simulink model "DesignTemperatureControlForDataCenter"  (R2025b)
settings: Solver=daessc  StartTime=0.0  StopTime=3600*4  FixedStep=0.5  MaxStep=1  RelTol=1e-3  AbsTol=1e-3
PreLoadFcn:
  | if ~exist("modelParam")
  |     setDefaultParameters;
  | end
undefined symbols (not defined in the file or in its folder): DiscIntNeverNeededParam, modelParam, value
libraries: fl_lib x78, nesl_utility x18, SimscapeFluids_lib x11, datacenter_lib x9, simulink_extras x4, slpidlib x2
(part 2 of 3)

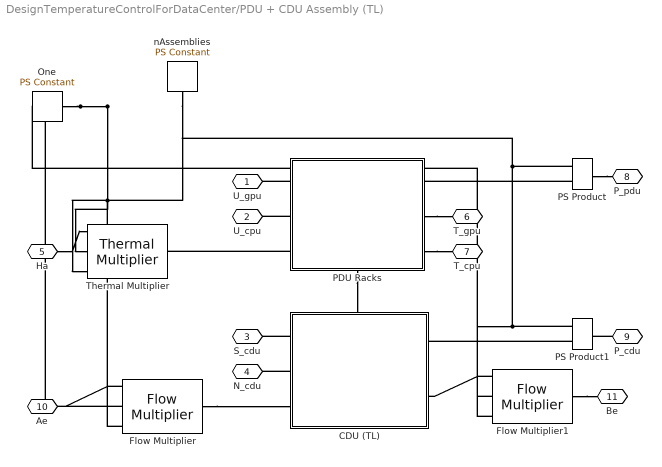
== system DesignTemperatureControlForDataCenter/PDU + CDU Assembly (TL) ==
  CDU (TL) : Subsystem  mask{extFluidMdot=extFluidMdot, extFluidPrDrop=extFluidPrDrop, extFluidVol=extFluidVol, extFluidPipeArea=extFluidPipeArea, intFluidMdot=intFluidMdot, intFluidPrDrop=intFluidPrDrop, intFluidVol=intFluidVol, intFluidPipeArea=intFluidPipeArea, spDissipationTbl=spDissipationTbl, effPipeLen=effPipeLen, pumpCapacityVec=pumpCapacityVec, pumpRefHeadVec=pumpRefHeadVec, pumpRefBrkPowVec=pumpRefBrkPowVec, pumpEff=pumpEff, nPumps=nPumps, speedLimFactor=speedLimFactor, pumpNominalRPM=pumpNominalRPM, pumpImpellerDiaFactor=pumpImpellerDiaFactor, iniT=initialT, iniP=initialP, refT=refT, refP=refP, refDensity=refDensity}
      mask prompts: extFluidMdot "External liquid loop mass flow rate vector (kg/s)"; extFluidPrDrop "External liquid loop pressure drop vector (kPa)"; extFluidVol "External liquid volume in heat exchanger (m^3)"; extFluidPipeArea "External liquid loop pipe cross-sectional area (m^2)"; intFluidMdot "Internal liquid loop mass flow rate vector (kg/s)"; intFluidPrDrop "Internal liquid loop pressure drop vector (kPa)"; intFluidVol "Internal liquid volume in heat exchanger (m^3)"; intFluidPipeArea "Internal liquid loop pipe cross-sectional area (m^2)"; spDissipationTbl "Specific dissipation table, SD[mdot_int,mdot_ext] (kW/K)"; effPipeLen "Effective pipe length for rack cooling (m)"; pumpCapacityVec "Reference capacity vector for each pump (m^3/s)"; pumpRefHeadVec "Reference head vector for each pump (m)"; pumpRefBrkPowVec "Reference brake power vector (kW)"; pumpEff "Electrical efficiency vector, 0-1 (-)"; nPumps "Total number of pumps (-)"; speedLimFactor "Pump speed upper limit factor (-)"; pumpNominalRPM "Pump nominal rating (rpm)"; pumpImpellerDiaFactor "Impeller diameter scale factor (-)"; iniT "Initial temperature (K)"; iniP "Initial pressure (MPa)"; refT "Reference flow temperature (K)"; refP "Reference flow pressure (MPa)"; refDensity "Reference density for internal liquid (kg/m^3)"
      settings: CopyFcn=set_param(gcbh,'LinkStatus','none');  PortSchema="{\"entries\":[{\"content\":{\"sides\":[{\"content\":{\"connectorIds\":[\"LConn1\",\"LConn2\",\"LConn3\"]},\"type\":\"ConnectorPlacement.EquallySpacedRectSide\",\"uuid\":\"dd9276e8-a048-49df-a05c-f18b45aafce3\"},{\"content\":{\"connectorIds\":[\"RConn1\",\"RConn2\"],\"side\":\"RIGHT\"},\"type\":\"ConnectorPlacement.EquallySpacedRectSide\",\"uuid\":\"f4cbe01b-cfd4-4d60-aff7-a07955033ed5\"},{\"content\":{\"connectorIds\":[\"LConn4\"],\"side\":\"TOP\"},\"type\":\"ConnectorPlacement.EquallySpacedRectSide\",\"uuid\":\"ad27df56-4241-452c-8570-6a66062dd2f2\"}]},\"type\":\"ConnectorPlacement.EquallySpacedConnector\",\"uuid\":\"0333b5f9-1896-45e0-922d-790b0e5dd980\"}],\"packageUris\":[\"http://schema.mathworks.com/mf0/Connector/R2020b\"],\"version\":\"1.0\"}"
      mask Help: web("DocumentationCDUTL.html")
      mask DialogControl Container5 Prompt: Heat Exchanger
      mask DialogControl Container8 Prompt: Set External Fluid Properties
      mask DialogControl Container7 Prompt: Set Internal Fluid Properties
      mask DialogControl Container9 Prompt: Heat Transfer
      mask DialogControl Container6 Prompt: Pumps
      mask DialogControl Container4 Prompt: Initial Conditions
      mask Display: image('icon_CDUthermalLiquid.png');
  Flow Multiplier : datacenter_lib/Flow Multiplier
      settings: InternalSimscapePortConfiguration="{\"Bottom\":[],\"Left\":[{\"id\":\"A\",\"label\":\"A\",\"type\":\"foundation.thermal_liquid.thermal_liquid\"}],\"Right\":[{\"id\":\"B\",\"label\":\"B\",\"type\":\"foundation.thermal_liquid.thermal_liquid\"}],\"Top\":[{\"id\":\"Na\",\"label\":\"Na\",\"type\":\"input\"},{\"id\":\"Nb\",\"label\":\"Nb\",\"type\":\"input\"}]}"
  Flow Multiplier1 : datacenter_lib/Flow Multiplier
      settings: InternalSimscapePortConfiguration="{\"Bottom\":[],\"Left\":[{\"id\":\"A\",\"label\":\"A\",\"type\":\"foundation.thermal_liquid.thermal_liquid\"}],\"Right\":[{\"id\":\"B\",\"label\":\"B\",\"type\":\"foundation.thermal_liquid.thermal_liquid\"}],\"Top\":[{\"id\":\"Na\",\"label\":\"Na\",\"type\":\"input\"},{\"id\":\"Nb\",\"label\":\"Nb\",\"type\":\"input\"}]}"
  One : fl_lib/Physical Signals/Sources/PS Constant  constant=1
  PDU Racks : Subsystem  mask{nTrays=nTrays, nRacks=nRacks, trayMass=trayMass, trayCp=trayCp, trayThermalR=trayThermalR, nGPU=nGPU, gpuTDPperDie=gpuTDPperDie, gpuIdlePower=gpuIdlePower, gpuHBMpower=gpuHBMpower, gpuExponent=gpuExponent, gpuHBMutil=gpuHBMutil, gpuLeakage=gpuLeakage, gpuNominalDieT=gpuNominalDieT, gpuDieThermalC=gpuDieThermalC, gpuHeatSinkR=gpuHeatSinkR, gpuSurfArea=gpuSurfArea, gpuAmbientR=gpuAmbientR, nCPU=nCPU, cpuTDPperSocket=cpuTDPperSocket, cpuIdlePower=cpuIdlePower, cpuExponent=cpuExponent, cpuLeakage=cpuLeakage, cpuNominalDieT=cpuNominalDieT, cpuDieThermalC=cpuDieThermalC, cpuHeatSinkR=cpuHeatSinkR, cpuSurfArea=cpuSurfArea, cpuAmbientR=cpuAmbientR, initialT=initialT, htc=htc}
      mask prompts: nTrays "Number of IT trays per rack (-)"; nRacks "Number of racks (-)"; trayMass "Tray mass (kg)"; trayCp "Tray specific heat capacity (J/kg*K)"; trayThermalR "Tray to external thermal resistance (K/W)"; nGPU "Number of GPU per tray (-)"; gpuTDPperDie "GPU TDP per die (W)"; gpuIdlePower "GPU idle power (W)"; gpuHBMpower "HBM power per GPU (W)"; gpuExponent "GPU power utilization exponent (-)"; gpuHBMutil "HBM utilization as fraction of compute utilization (-)"; gpuLeakage "Leakage increase per K above nominal temperature (W/K)"; gpuNominalDieT "Nominal die temperature at TDP (K)"; gpuDieThermalC "GPU die thermal capacitance (J/K)"; gpuHeatSinkR "GPU die-heat-sink thermal resistance (K/W)"; gpuSurfArea "Surface area per die for ambient heat transfer (m^2)"; gpuAmbientR "GPU die-ambient thermal resistance (K/W)"; nCPU "Number of CPU per tray (-)"; cpuTDPperSocket "CPU TDP per socket (W)"; cpuIdlePower "CPU idle power per socket (W)"; cpuExponent "CPU power utilization exponent (-)"; cpuLeakage "Leakage increase per K above nominal temperature (W/K)"; cpuNominalDieT "Nominal die temperature at TDP (K)"; cpuDieThermalC "CPU die thermal capacitance (J/K)"; cpuHeatSinkR "CPU die-heat-sink thermal resistance (K/W)"; cpuSurfArea "Surface area per die for ambient heat transfer (m^2)"; cpuAmbientR "CPU die-ambient thermal resistance (K/W)"; initialT "Initial temperature (K)"; htc "Heat transfer coefficient to ambient (W/m^2.K)"
      settings: CopyFcn=set_param(gcbh,'LinkStatus','none');  PortSchema="{\"entries\":[{\"content\":{\"sides\":[{\"content\":{\"connectorIds\":[\"LConn1\",\"LConn2\",\"LConn3\"]},\"type\":\"ConnectorPlacement.EquallySpacedRectSide\",\"uuid\":\"1a9a884a-dab1-4495-bf62-c6b2de6c1039\"},{\"content\":{\"connectorIds\":[\"RConn1\",\"RConn2\",\"RConn3\"],\"side\":\"RIGHT\"},\"type\":\"ConnectorPlacement.EquallySpacedRectSide\",\"uuid\":\"05c53434-51c1-4fee-b885-c321dcda8b6b\"},{\"content\":{\"side\":\"TOP\"},\"type\":\"ConnectorPlacement.EquallySpacedRectSide\",\"uuid\":\"c7b5c534-d596-4858-a133-27f005e6c9d4\"},{\"content\":{\"connectorIds\":[\"RConn4\"],\"side\":\"BOTTOM\"},\"type\":\"ConnectorPlacement.EquallySpacedRectSide\",\"uuid\":\"693f3c99-4296-4d86-bfcc-da753d3e576f\"}]},\"type\":\"ConnectorPlacement.EquallySpacedConnector\",\"uuid\":\"ed91c467-c4d0-403f-af16-bac0257594fd\"}],\"packageUris\":[\"http://schema.mathworks.com/mf0/Connector/R2020b\"],\"version\":\"1.0\"}"
      mask Help: web("DocumentationPDURacks.html")
      mask DialogControl Container10 Prompt: PDU Racks
      mask DialogControl getRatingButton Prompt: Get Rating
      mask DialogControl Container9 Prompt: IT Tray
      mask DialogControl Container6 Prompt: GPU
      mask DialogControl Container7 Prompt: CPU
      mask DialogControl Container8 Prompt: Initial Conditions
      mask Display: image('icon_PDURacks.png');
  PS Product : fl_lib/Physical Signals/Functions/PS Product
  PS Product1 : fl_lib/Physical Signals/Functions/PS Product
  Thermal Multiplier : datacenter_lib/Thermal Multiplier
      settings: InternalSimscapePortConfiguration="{\"Bottom\":[],\"Left\":[{\"id\":\"A\",\"label\":\"A\",\"type\":\"foundation.thermal.thermal\"}],\"Right\":[{\"id\":\"B\",\"label\":\"B\",\"type\":\"foundation.thermal.thermal\"}],\"Top\":[{\"id\":\"Na\",\"label\":\"Na\",\"type\":\"input\"},{\"id\":\"Nb\",\"label\":\"Nb\",\"type\":\"input\"}]}"
  nAssemblies : fl_lib/Physical Signals/Sources/PS Constant  constant=nAssembly
  U_gpu : PMIOPort  Side=Left
  U_cpu : PMIOPort  Port=2  Side=Left
  S_cdu : PMIOPort  Port=3  Side=Left
  N_cdu : PMIOPort  Port=4  Side=Left
  Ha : PMIOPort  Port=5  Side=Left
  T_gpu : PMIOPort  Port=6  Side=Right
  T_cpu : PMIOPort  Port=7  Side=Right
  P_pdu : PMIOPort  Port=8  Side=Right
  P_cdu : PMIOPort  Port=9  Side=Right
  Ae : PMIOPort  Port=10  Side=Right
  Be : PMIOPort  Port=11  Side=Right
  connections:
  P_cdu/RConn1 -- PS Product1/RConn1
  PS Product1/LConn2 -- CDU (TL)/RConn1
  PS Product/RConn1 -- P_pdu/RConn1
  PS Product/LConn2 -- PDU Racks/RConn1
  Flow Multiplier/LConn3 -- Thermal Multiplier/LConn3 -- PS Product/LConn1 -- Flow Multiplier1/LConn2 -- PS Product1/LConn1 -- nAssemblies/RConn1
  Thermal Multiplier/LConn2 -- Flow Multiplier1/LConn3 -- Flow Multiplier/LConn2 -- One/RConn1
  Flow Multiplier1/LConn1 -- CDU (TL)/RConn2
  Flow Multiplier1/RConn1 -- Be/RConn1
  Flow Multiplier/RConn1 -- CDU (TL)/LConn3
  Flow Multiplier/LConn1 -- Ae/RConn1
  Ha/RConn1 -- Thermal Multiplier/LConn1
  PDU Racks/LConn3 -- Thermal Multiplier/RConn1
  CDU (TL)/LConn1 -- S_cdu/RConn1
  PDU Racks/LConn1 -- U_gpu/RConn1
  PDU Racks/RConn2 -- T_gpu/RConn1
  CDU (TL)/LConn2 -- N_cdu/RConn1
  PDU Racks/LConn2 -- U_cpu/RConn1
  PDU Racks/RConn3 -- T_cpu/RConn1
  PDU Racks/RConn4 -- CDU (TL)/LConn4

== system DesignTemperatureControlForDataCenter/Pipe ==
  CDU External Water : SimscapeFluids_lib/Thermal Liquid/Utilities/Thermal Liquid Properties (TL)  fluid_list=fluids.thermal_liquid.utilities.enum.thermal_liquid_fluid_list.water  concentration_param_EG=fluids.thermal_liquid.utilities.enum.thermal_liquid_concentration.volume_fraction  concentration_param_PG=fluids.thermal_liquid.utilities.enum.thermal_liquid_concentration.volume_fraction  c_mass_SW=3.5e-3  c_mass_EG=0.1  c_mass_PG=0.1  c_mass_GL=0.1  c_vol_EG=0.1  c_vol_PG=0.1  beta_const_EG=2.1791 GPa  beta_const_PG=2.1791 GPa  beta_const_GL=2.1791 GPa  p_min_EG=0.01 MPa  p_min_PG=0.01 MPa  p_min_GL=0.01 MPa  p_max_EG=50 MPa  p_max_PG=50 MPa  p_max_GL=50 MPa  p_atm=0.101325 MPa  properties_range_check=simscape.enum.assert.action.error
  Perfect Insulator2 : fl_lib/Thermal/Thermal Elements/Perfect Insulator  T_specify=off  T_priority=None  T=293.15 K  T_nominal_specify=off  T_nominal_value=1  T_nominal_unit=K
  Pipe (TL)1 : fl_lib/Thermal Liquid/Elements/Pipe (TL)  length=.1 m  area=0.01*10 m^2  Dh=sqrt((4/pi)*0.01*10) m  length_add=1 m  roughness=15e-6 m  Re_lam=2000  Re_tur=4000  shape_factor=64  Nu_lam=3.66  dynamic_compressibility=true  inertia=false  p0=0.101325 MPa  T0="max(274,value(modelParam.WetBulbT ,\"K\")) K"  mdot0=0 kg/s  p_nominal=0.101325 MPa  T_nominal=293.15 K
  A : PMIOPort  Side=Left
  B : PMIOPort  Port=2  Side=Right
  connections:
  Perfect Insulator2/LConn1 -- Pipe (TL)1/LConn2
  A/RConn1 -- Pipe (TL)1/LConn1
  B/RConn1 -- CDU External Water/RConn1 -- Pipe (TL)1/RConn1

== system DesignTemperatureControlForDataCenter/Pipe  ==
  Cooling Tower Water : SimscapeFluids_lib/Thermal Liquid/Utilities/Thermal Liquid Properties (TL)  fluid_list=fluids.thermal_liquid.utilities.enum.thermal_liquid_fluid_list.water  concentration_param_EG=fluids.thermal_liquid.utilities.enum.thermal_liquid_concentration.volume_fraction  concentration_param_PG=fluids.thermal_liquid.utilities.enum.thermal_liquid_concentration.volume_fraction  c_mass_SW=3.5e-3  c_mass_EG=0.1  c_mass_PG=0.1  c_mass_GL=0.1  c_vol_EG=0.1  c_vol_PG=0.1  beta_const_EG=2.1791 GPa  beta_const_PG=2.1791 GPa  beta_const_GL=2.1791 GPa  p_min_EG=0.01 MPa  p_min_PG=0.01 MPa  p_min_GL=0.01 MPa  p_max_EG=50 MPa  p_max_PG=50 MPa  p_max_GL=50 MPa  p_atm=0.101325 MPa  properties_range_check=simscape.enum.assert.action.error
  Perfect Insulator3 : fl_lib/Thermal/Thermal Elements/Perfect Insulator  T_specify=off  T_priority=None  T=293.15 K  T_nominal_specify=off  T_nominal_value=1  T_nominal_unit=K
  Pipe (TL) : fl_lib/Thermal Liquid/Elements/Pipe (TL)  length=.1 m  area=0.01*10 m^2  Dh=sqrt((4/pi)*0.01*10) m  length_add=1 m  roughness=15e-6 m  Re_lam=2000  Re_tur=4000  shape_factor=64  Nu_lam=3.66  dynamic_compressibility=true  inertia=false  p0=0.101325 MPa  T0="max(274,value(modelParam.WetBulbT ,\"K\")) K"  mdot0=0 kg/s  p_nominal=0.101325 MPa  T_nominal=293.15 K
  A : PMIOPort  Side=Left
  B : PMIOPort  Port=2  Side=Right
  connections:
  Perfect Insulator3/LConn1 -- Pipe (TL)/LConn2
  Pipe (TL)/RConn1 -- Cooling Tower Water/RConn1 -- B/RConn1
  Pipe (TL)/LConn1 -- A/RConn1

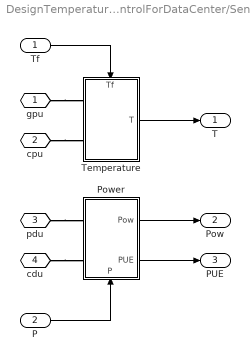
== system DesignTemperatureControlForDataCenter/Sensor ==
  Tf : Inport
  P : Inport  Port=2
  Power : Subsystem
      settings: PortSchema="{\"entries\":[{\"content\":{\"sides\":[{\"content\":{\"connectorIds\":[\"LConn1\",\"LConn2\"]},\"type\":\"ConnectorPlacement.EquallySpacedRectSide\",\"uuid\":\"9331510c-a4eb-4ecd-92c7-a7bb9d97a600\"},{\"content\":{\"connectorIds\":[\"Out1\",\"Out2\"],\"side\":\"RIGHT\"},\"type\":\"ConnectorPlacement.EquallySpacedRectSide\",\"uuid\":\"a10f6118-0032-4cdc-99b8-d09e72885979\"},{\"content\":{\"side\":\"TOP\"},\"type\":\"ConnectorPlacement.EquallySpacedRectSide\",\"uuid\":\"0f2ace20-053e-4299-9751-41cfaf8e15c6\"},{\"content\":{\"connectorIds\":[\"In1\"],\"side\":\"BOTTOM\"},\"type\":\"ConnectorPlacement.EquallySpacedRectSide\",\"uuid\":\"a9d7e431-b1c5-4489-9883-492d0aaca8bd\"}]},\"type\":\"ConnectorPlacement.EquallySpacedConnector\",\"uuid\":\"b3630bca-808a-4a4c-ac99-f11c77996374\"}],\"packageUris\":[\"http://schema.mathworks.com/mf0/Connector/R2020b\"],\"version\":\"1.0\"}"
  Temperature : Subsystem
      settings: PortSchema="{\"entries\":[{\"content\":{\"sides\":[{\"content\":{\"connectorIds\":[\"LConn1\",\"LConn2\"]},\"type\":\"ConnectorPlacement.EquallySpacedRectSide\",\"uuid\":\"38d708be-74dc-41fb-88b7-56224984dcb0\"},{\"content\":{\"connectorIds\":[\"Out1\"],\"side\":\"RIGHT\"},\"type\":\"ConnectorPlacement.EquallySpacedRectSide\",\"uuid\":\"bfba4674-b07b-4883-8c53-343b325b7582\"},{\"content\":{\"connectorIds\":[\"In1\"],\"side\":\"TOP\"},\"type\":\"ConnectorPlacement.EquallySpacedRectSide\",\"uuid\":\"d7238bf2-a2d8-47b2-91ac-f7562da6bea8\"},{\"content\":{\"side\":\"BOTTOM\"},\"type\":\"ConnectorPlacement.EquallySpacedRectSide\",\"uuid\":\"387bc73a-5c32-4219-8c37-7ff8149f1dcc\"}]},\"type\":\"ConnectorPlacement.EquallySpacedConnector\",\"uuid\":\"4e2610d2-3c00-4fd9-9aeb-66a40357b56e\"}],\"packageUris\":[\"http://schema.mathworks.com/mf0/Connector/R2020b\"],\"version\":\"1.0\"}"
  gpu : PMIOPort  Side=Left
  cpu : PMIOPort  Port=2  Side=Left
  pdu : PMIOPort  Port=3  Side=Left
  cdu : PMIOPort  Port=4  Side=Left
  T : Outport
  Pow : Outport  Port=2
  PUE : Outport  Port=3
  wires:
  Power/1(Pow) -> Pow/1
  Power/2(PUE) -> PUE/1
  Temperature/1(T) -> T/1
  Tf/1 -> Temperature/1(Tf)
  P/1 -> Power/1(P)
  connections:
  cpu/RConn1 -- Temperature/LConn2
  cdu/RConn1 -- Power/LConn2
  pdu/RConn1 -- Power/LConn1
  gpu/RConn1 -- Temperature/LConn1

== system DesignTemperatureControlForDataCenter/Subsystem ==
  " " : Inport
  Bus Selector : BusSelector  OutputSignals=CDU.S,CDU.N
  Simulink-PS Converter : nesl_utility/Simulink-PS Converter  PhysicalDomain=network_engine_domain  SubClassName=ps_input  LeftPortType=input  RightPortType=output  PseudoPeriodic=off  Frequencies=[]  NoiseDistribution=none  NoiseParameters=[]  Unit=1  AffineConversion=off  FilteringAndDerivatives=provide  SimscapeFilterOrder=1  InputFilterTimeConstant=0.001  UdotUserProvided=0
  Simulink-PS Converter1 : nesl_utility/Simulink-PS Converter  PhysicalDomain=network_engine_domain  SubClassName=ps_input  LeftPortType=input  RightPortType=output  PseudoPeriodic=off  Frequencies=[]  NoiseDistribution=none  NoiseParameters=[]  Unit=1  AffineConversion=off  FilteringAndDerivatives=provide  SimscapeFilterOrder=1  InputFilterTimeConstant=0.001  UdotUserProvided=0
  S : PMIOPort  Side=Right
  N : PMIOPort  Port=2  Side=Right
  wires:
  Bus Selector/1 -> Simulink-PS Converter/1  "<S>"
  Bus Selector/2 -> Simulink-PS Converter1/1  "<N>"
  " "/1 -> Bus Selector/1
  connections:
  Simulink-PS Converter1/RConn1 -- N/RConn1
  Simulink-PS Converter/RConn1 -- S/RConn1

== system DesignTemperatureControlForDataCenter/Subsystem1 ==
  " " : Inport
  Bus Selector : BusSelector  OutputSignals=Facilities.CDU External Pump
  Simulink-PS Converter : nesl_utility/Simulink-PS Converter  PhysicalDomain=network_engine_domain  SubClassName=ps_input  LeftPortType=input  RightPortType=output  PseudoPeriodic=off  Frequencies=[]  NoiseDistribution=none  NoiseParameters=[]  Unit=1  AffineConversion=off  FilteringAndDerivatives=provide  SimscapeFilterOrder=1  InputFilterTimeConstant=0.001  UdotUserProvided=0
  "  " : PMIOPort  Side=Right
  wires:
  Bus Selector/1 -> Simulink-PS Converter/1  "<CDU External Pump>"
  " "/1 -> Bus Selector/1
  connections:
  Simulink-PS Converter/RConn1 -- "  "/RConn1

== system DesignTemperatureControlForDataCenter/Subsystem2 ==
  " " : Inport
  Bus Selector : BusSelector  OutputSignals=Facilities.Tower pump
  Simulink-PS Converter : nesl_utility/Simulink-PS Converter  PhysicalDomain=network_engine_domain  SubClassName=ps_input  LeftPortType=input  RightPortType=output  PseudoPeriodic=off  Frequencies=[]  NoiseDistribution=none  NoiseParameters=[]  Unit=1  AffineConversion=off  FilteringAndDerivatives=provide  SimscapeFilterOrder=1  InputFilterTimeConstant=0.001  UdotUserProvided=0
  "  " : PMIOPort  Side=Right
  wires:
  Bus Selector/1 -> Simulink-PS Converter/1  "<Tower pump>"
  " "/1 -> Bus Selector/1
  connections:
  Simulink-PS Converter/RConn1 -- "  "/RConn1

== system DesignTemperatureControlForDataCenter/Subsystem3 ==
  "    " : Inport
  "   " : Inport  Port=2
  "  " : Inport  Port=3
  " " : Inport  Port=4
  Bus Creator : BusCreator  Inputs=4
  P : Outport
  wires:
  Bus Creator/1 -> P/1
  "   "/1 -> Bus Creator/3
  "  "/1 -> Bus Creator/2
  "    "/1 -> Bus Creator/1
  " "/1 -> Bus Creator/4

== system DesignTemperatureControlForDataCenter/Subsystem4 ==
  " " : Inport
  Bus Selector : BusSelector  OutputSignals=Facilities.Chiller
  Simulink-PS Converter : nesl_utility/Simulink-PS Converter  PhysicalDomain=network_engine_domain  SubClassName=ps_input  LeftPortType=input  RightPortType=output  PseudoPeriodic=off  Frequencies=[]  NoiseDistribution=none  NoiseParameters=[]  Unit=1  AffineConversion=off  FilteringAndDerivatives=provide  SimscapeFilterOrder=1  InputFilterTimeConstant=0.001  UdotUserProvided=0
  "  " : PMIOPort  Side=Right
  wires:
  Bus Selector/1 -> Simulink-PS Converter/1  "<Chiller>"
  " "/1 -> Bus Selector/1
  connections:
  Simulink-PS Converter/RConn1 -- "  "/RConn1

== system DesignTemperatureControlForDataCenter/Subsystem5 ==
  " " : Inport
  Bus Selector : BusSelector  OutputSignals=Facilities.Tower pump
  Simulink-PS Converter : nesl_utility/Simulink-PS Converter  PhysicalDomain=network_engine_domain  SubClassName=ps_input  LeftPortType=input  RightPortType=output  PseudoPeriodic=off  Frequencies=[]  NoiseDistribution=none  NoiseParameters=[]  Unit=1  AffineConversion=off  FilteringAndDerivatives=provide  SimscapeFilterOrder=1  InputFilterTimeConstant=0.001  UdotUserProvided=0
  "  " : PMIOPort  Side=Right
  wires:
  Bus Selector/1 -> Simulink-PS Converter/1  "<Tower pump>"
  " "/1 -> Bus Selector/1
  connections:
  Simulink-PS Converter/RConn1 -- "  "/RConn1

== system DesignTemperatureControlForDataCenter/Chiller/    ==
  PS-Simulink Converter4 : nesl_utility/PS-Simulink Converter  PhysicalDomain=network_engine_domain  SubClassName=ps_output  LeftPortType=input  RightPortType=output  PseudoPeriodic=off  Frequencies=[]  VectorFormat=inherit  Unit=inherit  AffineConversion=off
  Pressure & Temperature Sensor (TL) : fl_lib/Thermal Liquid/Sensors/Pressure & Temperature Sensor (TL)  reference=foundation.enum.MeasurementReference.absolute  pressure=false  pressure_spec=foundation.enum.PressureMeasementSpec.Absolute  temperature=true
      settings: InternalSimscapePortConfiguration="{\"Bottom\":[{\"id\":\"T\",\"label\":\"T\",\"type\":\"output\"}],\"Left\":[{\"id\":\"A\",\"label\":\"A\",\"type\":\"foundation.thermal_liquid.thermal_liquid\"}],\"Right\":[],\"Top\":[]}"
  " " : PMIOPort  Side=Right
  T : Outport
  wires:
  PS-Simulink Converter4/1 -> T/1
  connections:
  PS-Simulink Converter4/LConn1 -- Pressure & Temperature Sensor (TL)/RConn1
  Pressure & Temperature Sensor (TL)/LConn1 -- " "/RConn1

== system DesignTemperatureControlForDataCenter/Chiller/   1 ==
  PS-Simulink Converter4 : nesl_utility/PS-Simulink Converter  PhysicalDomain=network_engine_domain  SubClassName=ps_output  LeftPortType=input  RightPortType=output  PseudoPeriodic=off  Frequencies=[]  VectorFormat=inherit  Unit=inherit  AffineConversion=off
  Pressure & Temperature Sensor (TL) : fl_lib/Thermal Liquid/Sensors/Pressure & Temperature Sensor (TL)  reference=foundation.enum.MeasurementReference.absolute  pressure=false  pressure_spec=foundation.enum.PressureMeasementSpec.Absolute  temperature=true
      settings: InternalSimscapePortConfiguration="{\"Bottom\":[{\"id\":\"T\",\"label\":\"T\",\"type\":\"output\"}],\"Left\":[{\"id\":\"A\",\"label\":\"A\",\"type\":\"foundation.thermal_liquid.thermal_liquid\"}],\"Right\":[],\"Top\":[]}"
  " " : PMIOPort  Side=Right
  T : Outport
  wires:
  PS-Simulink Converter4/1 -> T/1
  connections:
  PS-Simulink Converter4/LConn1 -- Pressure & Temperature Sensor (TL)/RConn1
  Pressure & Temperature Sensor (TL)/LConn1 -- " "/RConn1

== system DesignTemperatureControlForDataCenter/Chiller/   2 ==
  PS-Simulink Converter4 : nesl_utility/PS-Simulink Converter  PhysicalDomain=network_engine_domain  SubClassName=ps_output  LeftPortType=input  RightPortType=output  PseudoPeriodic=off  Frequencies=[]  VectorFormat=inherit  Unit=inherit  AffineConversion=off
  Pressure & Temperature Sensor (TL) : fl_lib/Thermal Liquid/Sensors/Pressure & Temperature Sensor (TL)  reference=foundation.enum.MeasurementReference.absolute  pressure=false  pressure_spec=foundation.enum.PressureMeasementSpec.Absolute  temperature=true
      settings: InternalSimscapePortConfiguration="{\"Bottom\":[{\"id\":\"T\",\"label\":\"T\",\"type\":\"output\"}],\"Left\":[{\"id\":\"A\",\"label\":\"A\",\"type\":\"foundation.thermal_liquid.thermal_liquid\"}],\"Right\":[],\"Top\":[]}"
  " " : PMIOPort  Side=Right
  T : Outport
  wires:
  PS-Simulink Converter4/1 -> T/1
  connections:
  PS-Simulink Converter4/LConn1 -- Pressure & Temperature Sensor (TL)/RConn1
  Pressure & Temperature Sensor (TL)/LConn1 -- " "/RConn1

== system DesignTemperatureControlForDataCenter/Chiller/   3 ==
  PS-Simulink Converter4 : nesl_utility/PS-Simulink Converter  PhysicalDomain=network_engine_domain  SubClassName=ps_output  LeftPortType=input  RightPortType=output  PseudoPeriodic=off  Frequencies=[]  VectorFormat=inherit  Unit=inherit  AffineConversion=off
  Pressure & Temperature Sensor (TL) : fl_lib/Thermal Liquid/Sensors/Pressure & Temperature Sensor (TL)  reference=foundation.enum.MeasurementReference.absolute  pressure=false  pressure_spec=foundation.enum.PressureMeasementSpec.Absolute  temperature=true
      settings: InternalSimscapePortConfiguration="{\"Bottom\":[{\"id\":\"T\",\"label\":\"T\",\"type\":\"output\"}],\"Left\":[{\"id\":\"A\",\"label\":\"A\",\"type\":\"foundation.thermal_liquid.thermal_liquid\"}],\"Right\":[],\"Top\":[]}"
  " " : PMIOPort  Side=Left
  T : Outport
  wires:
  PS-Simulink Converter4/1 -> T/1
  connections:
  PS-Simulink Converter4/LConn1 -- Pressure & Temperature Sensor (TL)/RConn1
  Pressure & Temperature Sensor (TL)/LConn1 -- " "/RConn1

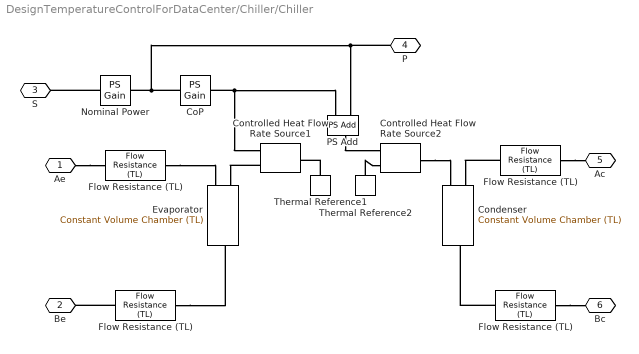
== system DesignTemperatureControlForDataCenter/Chiller/Chiller ==
  CoP : fl_lib/Physical Signals/Functions/PS Gain  gain=cop
  Condenser : fl_lib/Thermal Liquid/Elements/Constant Volume Chamber (TL)  volume=volume/2 m^3  num_ports=foundation.enum.num_ports.two  area_A=portArea m^2  area_B=portArea m^2  area_C=0.01 m^2  area_D=0.01 m^2  p_I_specify=on  p_I_priority=High  p_I=initialP MPa  p_I_nominal_specify=off  p_I_nominal_value=1  p_I_nominal_unit=MPa  T_I_specify=on  T_I_priority=High  T_I=initialT K  T_I_nominal_specify=off  T_I_nominal_value=1  T_I_nominal_unit=K  u_I_specify=off  u_I_priority=None  u_I=83.906 kJ/kg  u_I_nominal_specify=off  u_I_nominal_value=1  u_I_nominal_unit=kJ/kg  rho_I_specify=off  rho_I_priority=None  rho_I=998.21 kg/m^3  rho_I_nominal_specify=off  rho_I_nominal_value=1  rho_I_nominal_unit=kg/m^3
      settings: InternalSimscapePortConfiguration="{\"Bottom\":[],\"Left\":[{\"id\":\"A\",\"label\":\"A\",\"type\":\"foundation.thermal_liquid.thermal_liquid\"},{\"id\":\"H\",\"label\":\"H\",\"type\":\"foundation.thermal.thermal\"}],\"Right\":[{\"id\":\"B\",\"label\":\"B\",\"type\":\"foundation.thermal_liquid.thermal_liquid\"}],\"Top\":[]}"
  Controlled Heat Flow Rate Source1 : fl_lib/Thermal/Thermal Sources/Controlled Heat Flow Rate Source
  Controlled Heat Flow Rate Source2 : fl_lib/Thermal/Thermal Sources/Controlled Heat Flow Rate Source
  Evaporator : fl_lib/Thermal Liquid/Elements/Constant Volume Chamber (TL)  volume=volume/2 m^3  num_ports=foundation.enum.num_ports.two  area_A=portArea m^2  area_B=portArea m^2  area_C=0.01 m^2  area_D=0.01 m^2  p_I_specify=on  p_I_priority=High  p_I=3*initialP MPa  p_I_nominal_specify=off  p_I_nominal_value=1  p_I_nominal_unit=MPa  T_I_specify=on  T_I_priority=High  T_I=initialT K  T_I_nominal_specify=off  T_I_nominal_value=1  T_I_nominal_unit=K  u_I_specify=off  u_I_priority=None  u_I=83.906 kJ/kg  u_I_nominal_specify=off  u_I_nominal_value=1  u_I_nominal_unit=kJ/kg  rho_I_specify=off  rho_I_priority=None  rho_I=998.21 kg/m^3  rho_I_nominal_specify=off  rho_I_nominal_value=1  rho_I_nominal_unit=kg/m^3
      settings: InternalSimscapePortConfiguration="{\"Bottom\":[],\"Left\":[{\"id\":\"A\",\"label\":\"A\",\"type\":\"foundation.thermal_liquid.thermal_liquid\"},{\"id\":\"H\",\"label\":\"H\",\"type\":\"foundation.thermal.thermal\"}],\"Right\":[{\"id\":\"B\",\"label\":\"B\",\"type\":\"foundation.thermal_liquid.thermal_liquid\"}],\"Top\":[]}"
  Flow Resistance (TL) : fl_lib/Thermal Liquid/Elements/Flow Resistance (TL)  delta_p_nominal=nominalPrDrop/2 MPa  mdot_nominal=nominalFlowrate kg/s  area=portArea m^2  laminar_fraction=1e-3
  "Flow Resistance (TL) " : fl_lib/Thermal Liquid/Elements/Flow Resistance (TL)  delta_p_nominal=nominalPrDrop/2 MPa  mdot_nominal=nominalFlowrate kg/s  area=portArea m^2  laminar_fraction=1e-3
  "Flow Resistance (TL)  " : fl_lib/Thermal Liquid/Elements/Flow Resistance (TL)  delta_p_nominal=nominalPrDrop/2 MPa  mdot_nominal=nominalFlowrate kg/s  area=portArea m^2  laminar_fraction=1e-3
  "Flow Resistance (TL)   " : fl_lib/Thermal Liquid/Elements/Flow Resistance (TL)  delta_p_nominal=nominalPrDrop/2 MPa  mdot_nominal=nominalFlowrate kg/s  area=portArea m^2  laminar_fraction=1e-3
  Nominal Power : fl_lib/Physical Signals/Functions/PS Gain  gain=nominalRating*1000 J/s
  PS Add : fl_lib/Physical Signals/Functions/PS Add
  Thermal Reference1 : fl_lib/Thermal/Thermal Elements/Thermal Reference
  Thermal Reference2 : fl_lib/Thermal/Thermal Elements/Thermal Reference
  Ae : PMIOPort  Side=Left
  Be : PMIOPort  Port=2  Side=Left
  S : PMIOPort  Port=3  Side=Left
  P : PMIOPort  Port=4  Side=Left
  Ac : PMIOPort  Port=5  Side=Right
  Bc : PMIOPort  Port=6  Side=Right
  connections:
  Thermal Reference1/LConn1 -- Controlled Heat Flow Rate Source1/LConn1
  "Flow Resistance (TL) "/RConn1 -- Evaporator/RConn1
  Ae/RConn1 -- Flow Resistance (TL)/LConn1
  Nominal Power/LConn1 -- S/RConn1
  "Flow Resistance (TL)  "/LConn1 -- Condenser/LConn1
  Controlled Heat Flow Rate Source1/RConn2 -- Evaporator/LConn2
  CoP/RConn1 -- Controlled Heat Flow Rate Source1/RConn1 -- PS Add/LConn2
  Thermal Reference2/LConn1 -- Controlled Heat Flow Rate Source2/RConn2
  Flow Resistance (TL)/RConn1 -- Evaporator/LConn1
  Controlled Heat Flow Rate Source2/LConn1 -- Condenser/LConn2
  "Flow Resistance (TL)  "/RConn1 -- Ac/RConn1
  P/RConn1 -- PS Add/LConn1 -- CoP/LConn1 -- Nominal Power/RConn1
  "Flow Resistance (TL) "/LConn1 -- Be/RConn1
  "Flow Resistance (TL)   "/RConn1 -- Bc/RConn1
  "Flow Resistance (TL)   "/LConn1 -- Condenser/RConn1
  PS Add/RConn1 -- Controlled Heat Flow Rate Source2/RConn1

== system DesignTemperatureControlForDataCenter/Chiller/Subsystem ==
  "    " : Inport
  "   " : Inport  Port=2
  " " : Inport  Port=3
  "  " : Inport  Port=4
  Bus Creator1 : BusCreator  Inputs=4
  T : Outport
  wires:
  "   "/1 -> Bus Creator1/3
  "  "/1 -> Bus Creator1/2
  Bus Creator1/1 -> T/1
  " "/1 -> Bus Creator1/1
  "    "/1 -> Bus Creator1/4

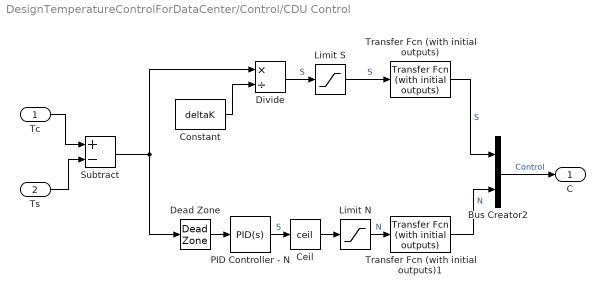
== system DesignTemperatureControlForDataCenter/Control/CDU Control ==
  "Tc " : Inport
  "Ts " : Inport  Port=2
  Bus Creator2 : BusCreator  Inputs=2
  Ceil : Rounding  Operator=ceil
  Constant : Constant  Value=deltaK
  Dead Zone : DeadZone  LowerValue=-deltaK/2  UpperValue=deltaK/2  ZeroCross=off
  Divide : Product  Inputs=*/
  Limit N : Saturate  UpperLimit=nPumps  LowerLimit=1  ZeroCross=off
  Limit S : Saturate  UpperLimit=1  LowerLimit=motorSpeed  ZeroCross=off
  PID Controller - N : slpidlib/PID Controller  Controller=PID  Form=Parallel  TimeDomain=Continuous-time  UseExternalTs=off  SampleTime=-1  IntegratorMethod=Forward Euler  FilterMethod=Forward Euler  ControllerParametersSource=internal  P=pidP  I=pidI  UseKiTs=off  D=pidD  UseExternalDerivativeSource=off  N=100  UseFilter=on  TunerSelectOption=Transfer Function Based (PID Tuner App)  ZeroCross=off  InitialConditionSource=internal  InitialConditionForIntegrator=1  InitialConditionForFilter=1  DifferentiatorICPrevScaledInput=0  ExternalReset=none  TrackingMode=off  Kt=1  LimitOutput=on  SatLimitsSource=internal  UpperSaturationLimit=nPumps  LowerSaturationLimit=0  LinearizeAsGain=on  AntiWindupMode=none  Kb=1  LimitIntegrator=off  UpperIntegratorSaturationLimit=inf  LowerIntegratorSaturationLimit=-inf  POutMin=[]  POutMax=[]  IOutMin=[]  IOutMax=[]  DOutMin=[]  DOutMax=[]  NOutMin=[]  NOutMax=[]  SumOutMin=[]  SumOutMax=[]  SaturationOutMin=[]  SaturationOutMax=[]  PParamMin=[]  PParamMax=[]  IParamMin=[]  IParamMax=[]  DParamMin=[]  DParamMax=[]  NParamMin=[]  NParamMax=[]  KbParamMin=[]  KbParamMax=[]  KtParamMin=[]  KtParamMax=[]  KbOutMin=[]  KbOutMax=[]  KtOutMin=[]  KtOutMax=[]  IntegratorOutMin=[]  IntegratorOutMax=[]  FilterOutMin=[]  FilterOutMax=[]  SumI1OutMin=[]  SumI1OutMax=[]  SumI2OutMin=[]  SumI2OutMax=[]  SumI3OutMin=[]  SumI3OutMax=[]  SumI4OutMin=[]  SumI4OutMax=[]  SumDOutMin=[]  SumDOutMax=[]  DifferentiatorOutMin=[]  DifferentiatorOutMax=[]  FilterDiffOutCoefMin=[]  FilterDiffOutCoefMax=[]  ReciprocalOutMin=[]  ReciprocalOutMax=[]  SumDenOutMin=[]  SumDenOutMax=[]  SumNumOutMin=[]  SumNumOutMax=[]  DivideOutMin=[]  DivideOutMax=[]  UdiffTsProdOutMin=[]  UdiffTsProdOutMax=[]  NTsProdOutMin=[]  NTsProdOutMax=[]  UintegralTsProdOutMin=[]  UintegralTsProdOutMax=[]  UngainTsProdOutMin=[]  UngainTsProdOutMax=[]  ClampingZeroOutDataTypeStr=Inherit: Inherit via back propagation  ClampingZeroOutMin=[]  ClampingZeroOutMax=[]  FilterDenConstantOutDataTypeStr=Inherit: Inherit via back propagation  FilterDenConstantOutMin=[]  FilterDenConstantOutMax=[]  PCopyOutDataTypeStr=Inherit: Inherit via back propagation  PCopyOutMin=[]  PCopyOutMax=[]  NCopyOutDataTypeStr=Inherit: Inherit via back propagation  NCopyOutMin=[]  NCopyOutMax=[]  IntegratorContinuousStateAttributes=''  IntegratorStateMustResolveToSignalObject=off  IntegratorRTWStateStorageClass=Auto  FilterContinuousStateAttributes=''  FilterStateMustResolveToSignalObject=off  FilterRTWStateStorageClass=Auto  ParallelPVariant=InternalParameters  IdealPVariant=Disabled  IVariant=InternalParameters  DVariant=InternalParameters  IntegratorVariant=Continuous  SatVariant=Enabled  AWVariant=Passthrough  PCopyVariant=Disabled  TRVariant=Disabled  FdbkBlocksVariant=Forward  IdealPFdbkVariant=Disabled  SatFdbkVariant=Disabled  DerivativeFilterVariant=ContFilter  NVariant=InternalParameters  NCopyVariant=Disabled  FilterICVariant=InternalICsFilter  IntegratorICVariant=InternalICs  ExternalResetVariant=Disabled  TRSumVariant=Passthrough  SumFdbkVariant=Disabled  SumVariant=Sum_PID  TsampFilterVariant=InternalTs  TsampNgainVariant=Passthrough  TsampIntegralVariant=Disabled_SignalSpec  ExternalSaturationOutDataTypeStr=Inherit: Same as second input  DerivativeSourceVariant=ErrorSignal  PreIntVariant=InternalPreInt
  Subtract : Sum  Inputs=+-
  Transfer Fcn (with initial outputs) : simulink_extras/Additional Linear/Transfer Fcn (with initial outputs)  N=[1]  D="[1  delaySec]"  Y0=1  U0=0
  Transfer Fcn (with initial outputs)1 : simulink_extras/Additional Linear/Transfer Fcn (with initial outputs)  N=[1]  D="[1  delaySec]"  Y0=1  U0=0
  C : Outport
  wires:
  Ceil/1 -> Limit N/1
  Bus Creator2/1 -> C/1  "Control"
  Dead Zone/1 -> PID Controller - N/1
  Subtract/1 -> Divide/1, Dead Zone/1
  Constant/1 -> Divide/2
  PID Controller - N/1 -> Ceil/1  "S"
  Limit N/1 -> Transfer Fcn (with initial outputs)1/1  "N"
  Divide/1 -> Limit S/1  "S"
  Limit S/1 -> Transfer Fcn (with initial outputs)/1  "S"
  "Tc "/1 -> Subtract/1
  "Ts "/1 -> Subtract/2
  Transfer Fcn (with initial outputs)/1 -> Bus Creator2/1  "S"
  Transfer Fcn (with initial outputs)1/1 -> Bus Creator2/2  "N"

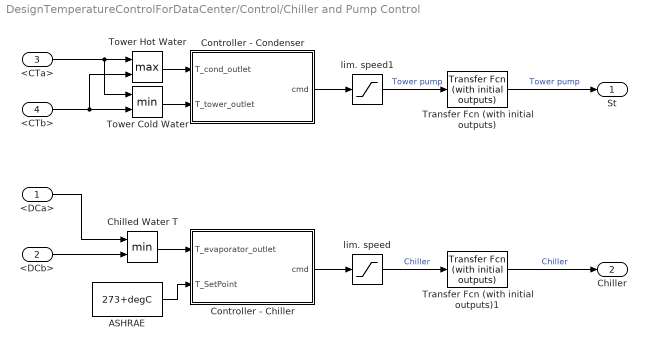
== system DesignTemperatureControlForDataCenter/Control/Chiller and Pump Control ==
  <DCa> : Inport
  <DCb> : Inport  Port=2
  <CTa> : Inport  Port=3
  <CTb> : Inport  Port=4
  ASHRAE : Constant  Value=273+degC
  Chilled Water T : MinMax  Inputs=2  ZeroCross=off
  Controller - Chiller : Subsystem
  Controller - Condenser : Subsystem
  Tower Cold Water : MinMax  Inputs=2  ZeroCross=off
  Tower Hot Water : MinMax  Function=max  Inputs=2  ZeroCross=off
  Transfer Fcn (with initial outputs) : simulink_extras/Additional Linear/Transfer Fcn (with initial outputs)  N=[1]  D="[1  delaySec]"  Y0=1  U0=0
  Transfer Fcn (with initial outputs)1 : simulink_extras/Additional Linear/Transfer Fcn (with initial outputs)  N=[1]  D="[1  delaySec]"  Y0=1  U0=0
  lim. speed : Saturate  UpperLimit=1  LowerLimit=0  ZeroCross=off
  lim. speed1 : Saturate  UpperLimit=1  LowerLimit=0  ZeroCross=off
  St : Outport
  Chiller : Outport  Port=2
  wires:
  <DCa>/1 -> Chilled Water T/1
  <CTb>/1 -> Tower Hot Water/2, Tower Cold Water/2
  <DCb>/1 -> Chilled Water T/2
  Tower Hot Water/1 -> Controller - Condenser/1(T_cond_outlet)
  Tower Cold Water/1 -> Controller - Condenser/2(T_tower_outlet)
  Chilled Water T/1 -> Controller - Chiller/1(T_evaporator_outlet)
  ASHRAE/1 -> Controller - Chiller/2(T_SetPoint)
  <CTa>/1 -> Tower Cold Water/1, Tower Hot Water/1
  Controller - Chiller/1(cmd) -> lim. speed/1
  Controller - Condenser/1(cmd) -> lim. speed1/1
  lim. speed1/1 -> Transfer Fcn (with initial outputs)/1  "Tower pump"
  lim. speed/1 -> Transfer Fcn (with initial outputs)1/1  "Chiller"
  Transfer Fcn (with initial outputs)/1 -> St/1  "Tower pump"
  Transfer Fcn (with initial outputs)1/1 -> Chiller/1  "Chiller"

== system DesignTemperatureControlForDataCenter/Control/Subsystem1 ==
  S : Inport
  Bus Selector : BusSelector  OutputSignals=S,N
  Product : Product
  Saturation : Saturate  UpperLimit=1  LowerLimit=0  ZeroCross=off
  P : Outport
  wires:
  Bus Selector/1 -> Product/1  "<S>"
  Product/1 -> Saturation/1
  Bus Selector/2 -> Product/2  "<N>"
  Saturation/1 -> P/1  "CDU External Pump"
  S/1 -> Bus Selector/1

== system DesignTemperatureControlForDataCenter/Cooling Tower /  ==
  Temperature Sensor : fl_lib/Thermal/Thermal Sensors/Temperature Sensor  temperature_measure=foundation.enum.MeasurementReference.difference
  Thermal Reference : fl_lib/Thermal/Thermal Elements/Thermal Reference
  " " : PMIOPort  Side=Left
  "   " : PMIOPort  Port=2  Side=Right
  connections:
  Temperature Sensor/RConn1 -- Thermal Reference/LConn1
  Temperature Sensor/RConn2 -- "   "/RConn1
  Temperature Sensor/LConn1 -- " "/RConn1

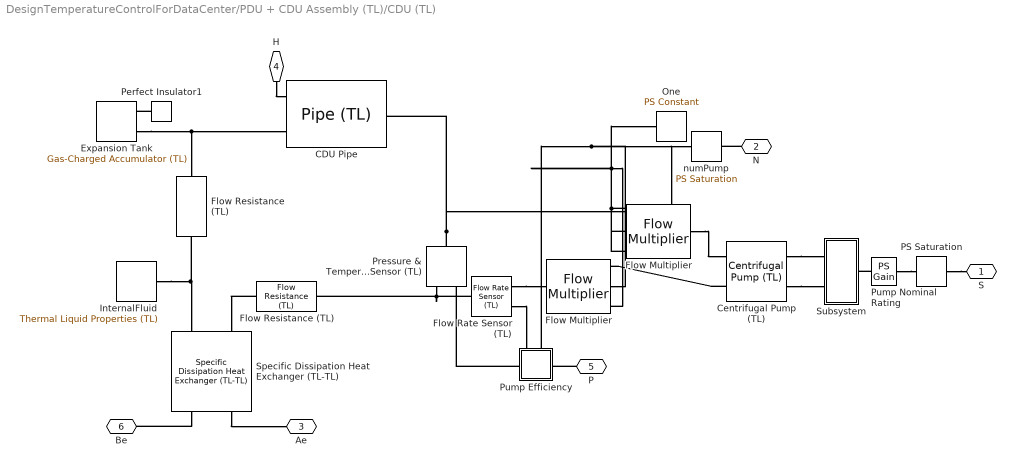
== system DesignTemperatureControlForDataCenter/PDU + CDU Assembly (TL)/CDU (TL) ==
  CDU Pipe : fl_lib/Thermal Liquid/Elements/Pipe (TL)  length=effPipeLen m  area=intFluidPipeArea m^2  Dh=sqrt(4*intFluidPipeArea/pi) m  length_add=1e-2 m  roughness=15e-6 m  Re_lam=2000  Re_tur=4000  shape_factor=64  Nu_lam=3.66  dynamic_compressibility=true  inertia=false  p0=iniP MPa  T0=iniT K  mdot0=0 kg/s  p_nominal=0.101325 MPa  T_nominal=293.15 K
  Centrifugal Pump (TL) : SimscapeFluids_lib/Thermal Liquid/Pumps & Motors/Centrifugal Pump (TL)  pump_parameterization=fluids.thermal_liquid.pumps_motors.enum.CentrifugalPumpParameterization.Table1D  capacity_ref_nominal=45 lpm  head_ref_nominal=40 m  power_ref_nominal=0.85 kW  head_ref_max=60 m  capacity_ref_max=80 lpm  omega_ref_analytic=1770 rpm  flow_rate_1D_TLU=pumpCapacityVec m^3/s  head_1D_TLU=pumpRefHeadVec m  power_1D_TLU=pumpRefBrkPowVec kW  omega_ref_1D=pumpNominalRPM rpm  rho_ref_1D=refDensity kg/m^3  omega_threshold_factor=1e-2  flow_rate_2D_TLU=[16.67, 23.33, 30, 40, 53.33, 60] lpm  omega_2D_TLU=[2450, 2800, 3150, 3500] rpm  head_2D_TLU=[25, 32.7, 42.5, 50; 24, 31.7, 41, 49; 22.7, 30.5, 39, 47.5; 20, 28, 36, 45; 15.7, 24, 32, 40; 12.5, 21, 29.5, 37.5] m  power_2D_TLU=[.28, .38, .5, .6; .31, .41, .55, .68; .33, .44, .6, .75; .36, .48, .65, .83; .38, .53, .72, .93; .39, .55, .75, .97] kW  rho_ref_2D=998.21 kg/m^3  diameter_ratio=pumpImpellerDiaFactor  mech_orientation=fluids.thermal_liquid.pumps_motors.enum.CentrifugalPumpMechOrientation.Positive  area=intFluidPipeArea/nPumps m^2  operation_check=simscape.enum.assert.action.none
      settings: InternalSimscapePortConfiguration="{\"Bottom\":[],\"Left\":[{\"id\":\"A\",\"label\":\"A\",\"type\":\"foundation.thermal_liquid.thermal_liquid\"},{\"id\":\"B\",\"label\":\"B\",\"type\":\"foundation.thermal_liquid.thermal_liquid\"}],\"Right\":[{\"id\":\"R\",\"label\":\"R\",\"type\":\"foundation.mechanical.rotational.rotational\"},{\"id\":\"C\",\"label\":\"C\",\"type\":\"foundation.mechanical.rotational.rotational\"}],\"Top\":[]}"
  Expansion Tank : SimscapeFluids_lib/Thermal Liquid/Tanks & Accumulators/Gas-Charged Accumulator (TL)  capacity=intFluidVol m^3  dead_volume=1e-3 m^3  p_precharge_gauge=iniP MPa  k_sh=1.4  area=intFluidPipeArea m^2  stiff_coeff=1e4 MPa/m^3  damping_coeff=1e4 MPa*s/m^6  liquid_volume_specify=on  liquid_volume_priority=None  liquid_volume=5e-3 m^3  liquid_volume_nominal_specify=off  liquid_volume_nominal_value=1  liquid_volume_nominal_unit=m^3  liquid_mass_specify=off  liquid_mass_priority=None  liquid_mass=5 kg  liquid_mass_nominal_specify=off  liquid_mass_nominal_value=1  liquid_mass_nominal_unit=kg  p_I_specify=on  p_I_priority=High  p_I=4*iniP MPa  p_I_nominal_specify=off  p_I_nominal_value=1  p_I_nominal_unit=MPa  T_I_specify=on  T_I_priority=High  T_I=iniT K  T_I_nominal_specify=off  T_I_nominal_value=1  T_I_nominal_unit=K
      settings: InternalSimscapePortConfiguration="{\"Bottom\":[],\"Left\":[],\"Right\":[{\"id\":\"A\",\"label\":\"A\",\"type\":\"foundation.thermal_liquid.thermal_liquid\"},{\"id\":\"H\",\"label\":\"H\",\"type\":\"foundation.thermal.thermal\"}],\"Top\":[]}"
  Flow Multiplier : datacenter_lib/Flow Multiplier
      settings: InternalSimscapePortConfiguration="{\"Bottom\":[],\"Left\":[{\"id\":\"A\",\"label\":\"A\",\"type\":\"foundation.thermal_liquid.thermal_liquid\"}],\"Right\":[{\"id\":\"B\",\"label\":\"B\",\"type\":\"foundation.thermal_liquid.thermal_liquid\"}],\"Top\":[{\"id\":\"Na\",\"label\":\"Na\",\"type\":\"input\"},{\"id\":\"Nb\",\"label\":\"Nb\",\"type\":\"input\"}]}"
  "Flow Multiplier " : datacenter_lib/Flow Multiplier
      settings: InternalSimscapePortConfiguration="{\"Bottom\":[],\"Left\":[{\"id\":\"A\",\"label\":\"A\",\"type\":\"foundation.thermal_liquid.thermal_liquid\"}],\"Right\":[{\"id\":\"B\",\"label\":\"B\",\"type\":\"foundation.thermal_liquid.thermal_liquid\"}],\"Top\":[{\"id\":\"Na\",\"label\":\"Na\",\"type\":\"input\"},{\"id\":\"Nb\",\"label\":\"Nb\",\"type\":\"input\"}]}"
  Flow Rate Sensor (TL) : fl_lib/Thermal Liquid/Sensors/Flow Rate Sensor (TL)  mass_flow_measure=false  volumetric_flow_measure=true  energy_flow_measure=false
      settings: InternalSimscapePortConfiguration="{\"Bottom\":[],\"Left\":[{\"id\":\"A\",\"label\":\"A\",\"type\":\"foundation.thermal_liquid.thermal_liquid\"}],\"Right\":[{\"id\":\"B\",\"label\":\"B\",\"type\":\"foundation.thermal_liquid.thermal_liquid\"},{\"id\":\"V\",\"label\":\"V\",\"type\":\"output\"}],\"Top\":[]}"
  Flow Resistance (TL) : fl_lib/Thermal Liquid/Elements/Flow Resistance (TL)  delta_p_nominal=0.1*min(intFluidPrDrop) kPa  mdot_nominal=min(intFluidMdot) kg/s  area=intFluidPipeArea m^2  laminar_fraction=1e-3
  "Flow Resistance (TL) " : fl_lib/Thermal Liquid/Elements/Flow Resistance (TL)  delta_p_nominal=0.1*min(intFluidPrDrop) kPa  mdot_nominal=min(intFluidMdot) kg/s  area=intFluidPipeArea m^2  laminar_fraction=1e-3
  InternalFluid : SimscapeFluids_lib/Thermal Liquid/Utilities/Thermal Liquid Properties (TL)  fluid_list=fluids.thermal_liquid.utilities.enum.thermal_liquid_fluid_list.water  concentration_param_EG=fluids.thermal_liquid.utilities.enum.thermal_liquid_concentration.volume_fraction  concentration_param_PG=fluids.thermal_liquid.utilities.enum.thermal_liquid_concentration.volume_fraction  c_mass_SW=3.5e-3  c_mass_EG=0.1  c_mass_PG=0.1  c_mass_GL=0.1  c_vol_EG=0.1  c_vol_PG=0.1  beta_const_EG=2.1791 GPa  beta_const_PG=2.1791 GPa  beta_const_GL=2.1791 GPa  p_min_EG=0.01 MPa  p_min_PG=0.01 MPa  p_min_GL=0.01 MPa  p_max_EG=50 MPa  p_max_PG=50 MPa  p_max_GL=50 MPa  p_atm=0.101325 MPa  properties_range_check=simscape.enum.assert.action.error
  One : fl_lib/Physical Signals/Sources/PS Constant  constant=1
  PS Saturation : fl_lib/Physical Signals/Nonlinear Operators/PS Saturation  upper_limit=speedLimFactor  lower_limit=0  ZeroCross=true
  Perfect Insulator1 : fl_lib/Thermal/Thermal Elements/Perfect Insulator  T_specify=off  T_priority=None  T=293.15 K  T_nominal_specify=off  T_nominal_value=1  T_nominal_unit=K
  Pressure & Temperature Sensor (TL) : fl_lib/Thermal Liquid/Sensors/Pressure & Temperature Sensor (TL)  reference=foundation.enum.MeasurementReference.difference  pressure=true  pressure_spec=foundation.enum.PressureMeasementSpec.Absolute  temperature=false
      settings: InternalSimscapePortConfiguration="{\"Bottom\":[],\"Left\":[{\"id\":\"A\",\"label\":\"A\",\"type\":\"foundation.thermal_liquid.thermal_liquid\"}],\"Right\":[{\"id\":\"B\",\"label\":\"B\",\"type\":\"foundation.thermal_liquid.thermal_liquid\"},{\"id\":\"P\",\"label\":\"P\",\"type\":\"output\"}],\"Top\":[]}"
  Pump Efficiency : Subsystem
      settings: PortSchema="{\"entries\":[{\"content\":{\"sides\":[{\"content\":{\"connectorIds\":[\"LConn1\"]},\"type\":\"ConnectorPlacement.EquallySpacedRectSide\",\"uuid\":\"7c880f53-79d7-4fc1-b853-6a19eeb267d6\"},{\"content\":{\"connectorIds\":[\"RConn1\"],\"side\":\"RIGHT\"},\"type\":\"ConnectorPlacement.EquallySpacedRectSide\",\"uuid\":\"ee796b5d-8f71-4c2c-8982-d65c9b09dfff\"},{\"content\":{\"connectorIds\":[\"LConn2\",\"LConn3\"],\"side\":\"TOP\"},\"type\":\"ConnectorPlacement.EquallySpacedRectSide\",\"uuid\":\"11e8f51e-a30e-473a-bd43-abeec225f5c9\"}]},\"type\":\"ConnectorPlacement.EquallySpacedConnector\",\"uuid\":\"3106b96b-5b56-4bfa-809a-5c3e3f25fbb5\"}],\"packageUris\":[\"http://schema.mathworks.com/mf0/Connector/R2020b\"],\"version\":\"1.0\"}"
  Pump Nominal Rating : fl_lib/Physical Signals/Functions/PS Gain  gain=pumpNominalRPM rpm
  Specific Dissipation Heat Exchanger (TL-TL) : SimscapeFluids_lib/Heat Exchangers/Thermal Liquid/Specific Dissipation Heat Exchanger (TL-TL)  mdot1_TLU=intFluidMdot kg/s  mdot2_TLU=extFluidMdot kg/s  SD_TLU=spDissipationTbl kW/K  Q_check=simscape.enum.assert.action.none  mdot_dp_TLU_1=intFluidMdot kg/s  p_diff_TLU_1=intFluidPrDrop-0.2*min(intFluidPrDrop) kPa  T_ref_in_1=refT K  p_ref_in_1=refP MPa  mdot_threshold_1=1e-3 kg/s  liquid_volume_1=intFluidVol m^3  area_1=intFluidPipeArea m^2  mdot_dp_TLU_2=extFluidMdot kg/s  p_diff_TLU_2=extFluidPrDrop kPa  T_ref_in_2=refT K  p_ref_in_2=refP MPa  mdot_threshold_2=1e-3 kg/s  liquid_volume_2=extFluidVol m^3  area_2=extFluidPipeArea m^2  dynamic_compressibility_1=true  T0_1=iniT K  p0_1=iniP MPa  T_nominal_1=293.15 K  p_nominal_1=0.101325 MPa  dynamic_compressibility_2=true  T0_2=iniT K  p0_2=iniP MPa  T_nominal_2=293.15 K  p_nominal_2=0.101325 MPa
      settings: InternalSimscapePortConfiguration="{\"Bottom\":[],\"Left\":[{\"id\":\"A1\",\"label\":\"A1\",\"type\":\"foundation.thermal_liquid.thermal_liquid\"},{\"id\":\"B1\",\"label\":\"B1\",\"type\":\"foundation.thermal_liquid.thermal_liquid\"}],\"Right\":[{\"id\":\"A2\",\"label\":\"A2\",\"type\":\"foundation.thermal_liquid.thermal_liquid\"},{\"id\":\"B2\",\"label\":\"B2\",\"type\":\"foundation.thermal_liquid.thermal_liquid\"}],\"Top\":[]}"
  Subsystem : Subsystem
  numPump : fl_lib/Physical Signals/Nonlinear Operators/PS Saturation  upper_limit=nPumps  lower_limit=0  ZeroCross=true
  S : PMIOPort  Side=Left
  N : PMIOPort  Port=2  Side=Left
  Ae : PMIOPort  Port=3  Side=Left
  H : PMIOPort  Port=4  Side=Left
  P : PMIOPort  Port=5  Side=Right
  Be : PMIOPort  Port=6  Side=Right
  connections:
  H/RConn1 -- CDU Pipe/LConn2
  Specific Dissipation Heat Exchanger (TL-TL)/RConn2 -- Be/RConn1
  Expansion Tank/RConn1 -- CDU Pipe/LConn1 -- Flow Resistance (TL)/LConn1
  Specific Dissipation Heat Exchanger (TL-TL)/RConn1 -- Ae/RConn1
  InternalFluid/RConn1 -- Specific Dissipation Heat Exchanger (TL-TL)/LConn2 -- Flow Resistance (TL)/RConn1
  Centrifugal Pump (TL)/RConn2 -- Subsystem/LConn2
  Centrifugal Pump (TL)/RConn1 -- Subsystem/LConn1
  Pump Nominal Rating/RConn1 -- Subsystem/RConn1
  Perfect Insulator1/LConn1 -- Expansion Tank/RConn2
  Pump Nominal Rating/LConn1 -- PS Saturation/RConn1
  PS Saturation/LConn1 -- S/RConn1
  "Flow Resistance (TL) "/RConn1 -- Specific Dissipation Heat Exchanger (TL-TL)/LConn1
  Pressure & Temperature Sensor (TL)/LConn1 -- CDU Pipe/RConn1 -- Flow Multiplier/LConn1
  Flow Multiplier/RConn1 -- Centrifugal Pump (TL)/LConn1
  Flow Rate Sensor (TL)/LConn1 -- "Flow Resistance (TL) "/LConn1 -- Pressure & Temperature Sensor (TL)/RConn1
  P/RConn1 -- Pump Efficiency/RConn1
  Flow Rate Sensor (TL)/RConn2 -- Pump Efficiency/LConn2
  Pump Efficiency/LConn1 -- Pressure & Temperature Sensor (TL)/RConn2
  N/RConn1 -- numPump/LConn1
  Centrifugal Pump (TL)/LConn2 -- "Flow Multiplier "/LConn1
  Flow Rate Sensor (TL)/RConn1 -- "Flow Multiplier "/RConn1
  Flow Multiplier/LConn3 -- Pump Efficiency/LConn3 -- "Flow Multiplier "/LConn2 -- numPump/RConn1
  Flow Multiplier/LConn2 -- "Flow Multiplier "/LConn3 -- One/RConn1
